simulink model "gm_sampleModel1839_sub_sub"  (R2023a)
settings: Solver=VariableStepAuto  StartTime=0.0  StopTime=10.0  RelTol=1e-3
libraries: hdlsllib x3, simulink x1
settings Model: Creator=user1  LastModifiedBy=user1
settings OptimizationCC: BlockReduction=off  ConditionallyExecuteInputs=off
settings DebuggingCC: InheritedTsInSrcMsg=none

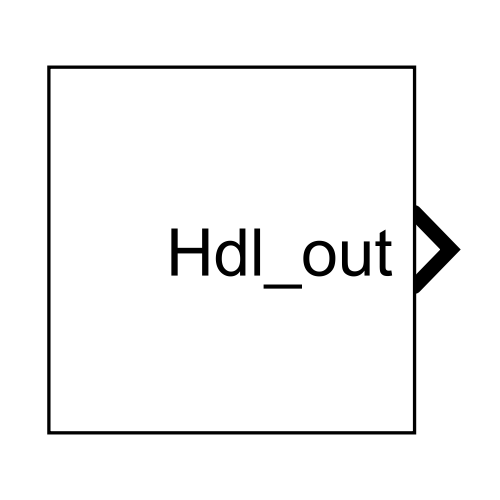
[thumbnail: Simulink's stored preview of the top-level diagram]
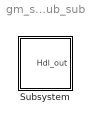
== system gm_sampleModel1839_sub_sub ==
  Subsystem : Subsystem

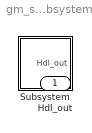
== system gm_sampleModel1839_sub_sub/Subsystem ==
  Subsystem : Subsystem
  Hdl_out : Outport  OutDataTypeStr=uint8

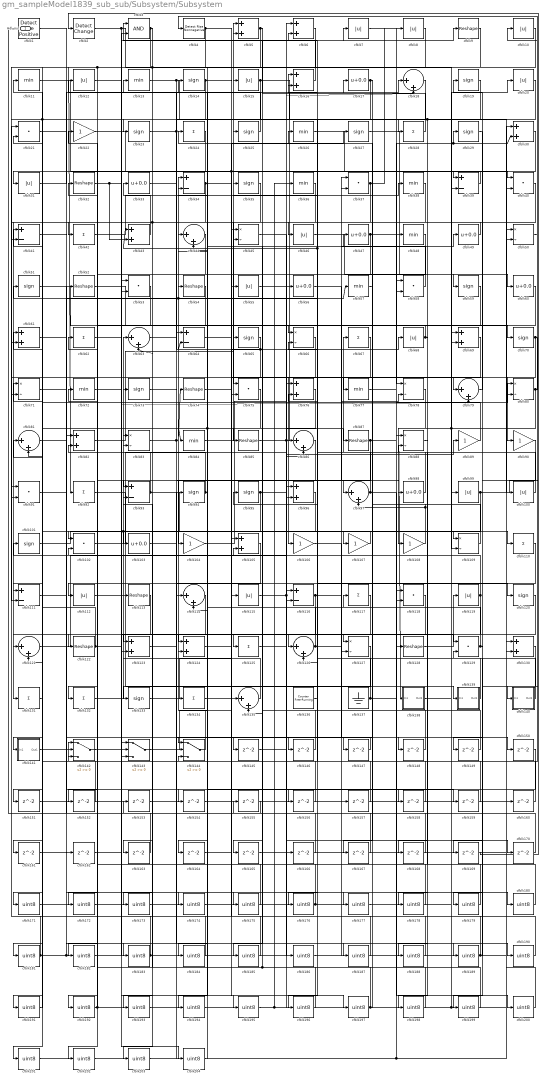
== system gm_sampleModel1839_sub_sub/Subsystem/Subsystem ==
  cfblk1 : hdlsllib/Logic and Bit Operations/Detect Rise Positive  vinit=0  OutDataTypeStr=uint8
  cfblk{7..8,10,12,15,20,31,46,55,68,99..100,112,115,119} (15 alike) : Abs  OutDataTypeStr=uint8  SaturateOnIntegerOverflow=off
  cfblk{14,19,23,25,27,29,35,51,59,65,70,73,94..95,101,120,133} (17 alike) : Signum
  cfblk{21,37,40,53,58,75,91,102,118,129} (10 alike) : DotProduct  OutDataTypeStr=uint8
  cfblk{17,33,47,49,56,60,98,103} (8 alike) : Bias  Bias=0.0  SaturateOnIntegerOverflow=off
  cfblk{22,89..90,104,106..108} (7 alike) : Gain  OutDataTypeStr=uint8
  cfblk{5..6,16,30,43,61,69,76,82,96,105,123..124,130} (14 alike) : Sum  OutDataTypeStr=uint8
  cfblk{45,50,66,71,78,80,83,88,109,127} (10 alike) : Product  Inputs=*/  OutDataTypeStr=uint8  RndMeth=Zero  SaturateOnIntegerOverflow=on
  cfblk{11,13,26,36,38,48,57,72,77,84} (10 alike) : MinMax  OutDataTypeStr=uint8
  cfblk{24,28,42,62,67,92,110,117,125,131..132,134} (12 alike) : Sum  Inputs=+  OutDataTypeStr=uint8
  cfblk{34,39,41,64,93,111,116} (7 alike) : Sum  Inputs=+-  OutDataTypeStr=uint8
  cfblk{9,32,52,54,74,85,87,113,122,128} (10 alike) : Reshape
  cfblk{18,44,63,79,81,86,97,114,121,126,135} (11 alike) : Sum  Inputs=|++  OutDataTypeStr=uint8
  cfblk136 : hdlsllib/Sources/Counter Free-Running  NumBits=16  tsamp=-1
  cfblk137 : Ground
  cfblk138 : Subsystem
      settings: LibrarySourceBlock=|
      | hdlsllib/Ports &
      | Subsystems/Subsystem
  cfblk139 : Subsystem
      settings: LibrarySourceBlock=|
      | hdlsllib/Ports &
      | Subsystems/Subsystem
  cfblk140 : Subsystem
      settings: LibrarySourceBlock=|
      | hdlsllib/Ports &
      | Subsystems/Subsystem
  cfblk141 : Subsystem
      settings: LibrarySourceBlock=|
      | hdlsllib/Ports &
      | Subsystems/Subsystem
  cfblk142 : Switch  OutDataTypeStr=uint8  SaturateOnIntegerOverflow=off  InputSameDT=off
  cfblk143 : Switch  OutDataTypeStr=uint8  SaturateOnIntegerOverflow=off  InputSameDT=off
  cfblk144 : Switch  OutDataTypeStr=uint8  SaturateOnIntegerOverflow=off  InputSameDT=off
  cfblk{145..170} (26 alike) : Delay  SampleTime=1
  cfblk{171..204} (34 alike) : DataTypeConversion  OutDataTypeStr=uint8  SaturateOnIntegerOverflow=off  RndMeth=Floor
  cfblk2 : simulink/Logic and Bit Operations/Detect Change  vinit=0  OutDataTypeStr=uint8
      settings: LibrarySourceBlock=|
      | hdlsllib/Logic and Bit
      | Operations/Detect
      | Change
  cfblk3 : Logic  AllPortsSameDT=off  OutDataTypeStr=boolean
  cfblk4 : hdlsllib/Logic and Bit Operations/Detect Rise Nonnegative  vinit=0  OutDataTypeStr=uint8
  Hdl_out : Outport  OutDataTypeStr=uint8
  wires:
  cfblk130/1 -> cfblk199/1
  cfblk128/1 -> cfblk119/1
  cfblk35/1 -> cfblk131/1
  cfblk70/1 -> cfblk140/1(In1), cfblk90/1
  cfblk126/1 -> cfblk78/2, cfblk101/1
  cfblk52/1 -> cfblk70/1
  cfblk21/1 -> cfblk183/1
  cfblk85/1 -> cfblk87/1, cfblk17/1
  cfblk68/1 -> cfblk168/1, cfblk66/1
  cfblk84/1 -> cfblk5/1
  cfblk40/1 -> cfblk75/1
  cfblk37/1 -> cfblk133/1, cfblk8/1
  cfblk22/1 -> cfblk39/1
  cfblk108/1 -> cfblk97/2, cfblk24/1
  cfblk115/1 -> cfblk170/1, cfblk18/2
  cfblk49/1 -> cfblk46/1
  cfblk50/1 -> cfblk4/1
  cfblk104/1 -> cfblk56/1
  cfblk95/1 -> cfblk89/1, cfblk103/1, cfblk111/1
  cfblk98/1 -> cfblk67/1
  cfblk144/1 -> cfblk34/1
  cfblk83/1 -> cfblk159/1, cfblk74/1
  cfblk4/1 -> cfblk180/1, cfblk173/1, cfblk42/1, cfblk92/1
  cfblk140/1(Out1) -> cfblk35/1
  cfblk16/1 -> cfblk3/1
  cfblk5/1 -> cfblk165/1, cfblk164/1
  cfblk132/1 -> cfblk63/1
  cfblk19/1 -> cfblk194/1, cfblk84/1
  cfblk87/1 -> cfblk104/1, cfblk30/2, cfblk29/1
  cfblk27/1 -> cfblk59/1
  cfblk72/1 -> cfblk195/1
  cfblk97/1 -> cfblk200/1, cfblk16/1
  cfblk92/1 -> cfblk139/1(In1)
  cfblk101/1 -> cfblk107/1
  cfblk66/1 -> cfblk85/1
  cfblk76/1 -> cfblk121/1
  cfblk73/1 -> cfblk120/1
  cfblk17/1 -> cfblk147/1, cfblk146/1
  cfblk42/1 -> cfblk38/1
  cfblk82/1 -> cfblk65/1
  cfblk135/1 -> cfblk73/1
  cfblk18/1 -> cfblk124/1
  cfblk133/1 -> cfblk55/1
  cfblk48/1 -> cfblk125/1
  cfblk109/1 -> cfblk25/1
  cfblk93/1 -> cfblk83/2, cfblk110/1
  cfblk69/1 -> cfblk111/2
  cfblk138/1(Out1) -> cfblk20/1
  cfblk65/1 -> cfblk91/2, cfblk64/2
  cfblk39/1 -> cfblk31/1
  cfblk116/1 -> cfblk143/3, cfblk49/1
  cfblk122/1 -> cfblk129/1, cfblk41/1
  cfblk36/1 -> cfblk41/2
  cfblk14/1 -> cfblk77/1, cfblk23/1
  cfblk47/1 -> cfblk152/1, cfblk80/2
  cfblk67/1 -> cfblk106/1
  cfblk43/1 -> cfblk33/1
  cfblk143/1 -> cfblk68/1
  cfblk64/1 -> cfblk126/1
  cfblk46/1 -> cfblk60/1
  cfblk59/1 -> cfblk123/1
  cfblk137/1 -> cfblk80/1, cfblk95/1
  cfblk6/1 -> cfblk144/1
  cfblk79/1 -> cfblk19/1
  cfblk119/1 -> cfblk161/1, cfblk83/1
  cfblk102/1 -> cfblk6/1
  cfblk94/1 -> cfblk44/2, cfblk32/1
  cfblk131/1 -> cfblk71/1
  cfblk99/1 -> cfblk191/1, cfblk142/1
  cfblk26/1 -> cfblk58/1
  cfblk51/1 -> cfblk116/1
  cfblk141/1(Out1) -> cfblk54/1, cfblk57/1
  cfblk80/1 -> cfblk10/1, cfblk109/2, cfblk138/1(In1)
  cfblk1/1 -> cfblk82/1
  cfblk25/1 -> cfblk13/1
  cfblk13/1 -> cfblk127/2, cfblk100/1
  cfblk3/1 -> cfblk203/1, cfblk61/2
  cfblk114/1 -> cfblk202/1
  cfblk81/1 -> cfblk189/1
  cfblk23/1 -> cfblk28/1, cfblk109/1
  cfblk139/1(Out1) -> cfblk51/1
  cfblk107/1 -> cfblk102/1
  cfblk32/1 -> cfblk43/2, cfblk127/1
  cfblk136/1 -> cfblk26/1
  cfblk38/1 -> cfblk132/1
  cfblk78/1 -> cfblk108/1
  cfblk96/1 -> cfblk135/2
  cfblk15/1 -> cfblk53/2, cfblk99/1
  cfblk11/1 -> cfblk78/1, cfblk115/1
  cfblk129/1 -> cfblk179/1, cfblk12/1
  cfblk121/1 -> cfblk96/2
  cfblk74/1 -> cfblk27/1
  cfblk134/1 -> cfblk197/1
  cfblk113/1 -> cfblk181/1
  cfblk7/1 -> cfblk40/1
  cfblk10/1 -> cfblk201/1, cfblk63/2
  cfblk86/1 -> cfblk192/1
  cfblk56/1 -> cfblk98/1
  cfblk55/1 -> cfblk7/1
  cfblk2/1 -> cfblk79/2, cfblk69/2
  cfblk117/1 -> cfblk176/1
  cfblk124/1 -> cfblk75/2
  cfblk33/1 -> cfblk97/1
  cfblk100/1 -> cfblk16/2, cfblk43/1
  cfblk31/1 -> cfblk15/1
  cfblk34/1 -> cfblk79/1, cfblk193/1, cfblk143/2
  cfblk63/1 -> cfblk18/1
  cfblk44/1 -> cfblk93/1
  cfblk20/1 -> cfblk188/1, cfblk141/1(In1), cfblk71/2
  cfblk8/1 -> cfblk122/1
  cfblk77/1 -> cfblk48/1
  cfblk58/1 -> cfblk14/1
  cfblk24/1 -> cfblk112/1
  cfblk89/1 -> cfblk61/1
  cfblk54/1 -> cfblk123/2
  cfblk28/1 -> cfblk5/2
  cfblk142/1 -> cfblk9/1
  cfblk111/1 -> cfblk52/1
  cfblk60/1 -> cfblk145/1
  cfblk145/1 -> cfblk116/2
  cfblk146/1 -> cfblk64/1
  cfblk147/1 -> cfblk144/2
  cfblk106/1 -> cfblk148/1
  cfblk148/1 -> cfblk66/2
  cfblk29/1 -> cfblk149/1
  cfblk149/1 -> cfblk102/2
  cfblk41/1 -> cfblk150/1
  cfblk75/1 -> cfblk151/1
  cfblk151/1 -> cfblk96/1
  cfblk152/1 -> cfblk121/2
  cfblk153/1 -> cfblk37/1
  cfblk12/1 -> cfblk154/1
  cfblk154/1 -> cfblk50/2
  cfblk155/1 -> cfblk1/1
  cfblk110/1 -> cfblk156/1
  cfblk156/1 -> cfblk34/2
  cfblk157/1 -> cfblk76/2
  cfblk91/1 -> cfblk158/1
  cfblk158/1 -> cfblk105/2
  cfblk159/1 -> cfblk126/2
  cfblk160/1 -> cfblk6/2
  cfblk161/1 -> cfblk3/2
  cfblk61/1 -> cfblk162/1
  cfblk162/1 -> cfblk143/1
  cfblk127/1 -> cfblk163/1
  cfblk163/1 -> cfblk142/3
  cfblk164/1 -> cfblk135/1
  cfblk165/1 -> cfblk30/1
  cfblk125/1 -> cfblk166/1
  cfblk166/1 -> cfblk82/2
  cfblk57/1 -> cfblk167/1
  cfblk167/1 -> cfblk142/2
  cfblk168/1 -> cfblk144/3
  cfblk90/1 -> cfblk169/1
  cfblk169/1 -> cfblk2/1
  cfblk170/1 -> cfblk11/1
  cfblk118/1 -> cfblk171/1
  cfblk171/1 -> cfblk94/1
  cfblk53/1 -> cfblk172/1
  cfblk172/1 -> cfblk118/1
  cfblk173/1 -> cfblk118/2
  cfblk62/1 -> cfblk174/1
  cfblk174/1 -> cfblk69/1
  cfblk103/1 -> cfblk175/1
  cfblk175/1 -> cfblk62/1
  cfblk176/1 -> cfblk58/2, cfblk44/1
  cfblk71/1 -> cfblk177/1
  cfblk177/1 -> cfblk117/1
  cfblk88/1 -> cfblk178/1
  cfblk178/1 -> cfblk153/1
  cfblk179/1 -> cfblk88/1
  cfblk180/1 -> cfblk88/2
  cfblk181/1 -> cfblk91/1, cfblk187/1, cfblk157/1
  cfblk105/1 -> cfblk182/1
  cfblk182/1 -> cfblk113/1
  cfblk183/1 -> cfblk50/1, cfblk53/1
  cfblk150/1 -> cfblk184/1
  cfblk184/1 -> cfblk21/1
  cfblk9/1 -> cfblk185/1
  cfblk185/1 -> cfblk21/2
  cfblk45/1 -> cfblk186/1
  cfblk186/1 -> cfblk37/2
  cfblk187/1 -> cfblk45/1
  cfblk188/1 -> cfblk45/2
  cfblk189/1 -> cfblk105/1, cfblk129/2
  cfblk123/1 -> cfblk190/1
  cfblk190/1 -> cfblk81/1
  cfblk191/1 -> cfblk81/2
  cfblk192/1 -> cfblk22/1, cfblk39/2, cfblk40/2
  cfblk193/1 -> cfblk86/1
  cfblk194/1 -> cfblk86/2
  cfblk195/1 -> cfblk36/1, cfblk76/1
  cfblk30/1 -> cfblk196/1
  cfblk196/1 -> cfblk72/1
  cfblk197/1 -> cfblk124/2, cfblk47/1
  cfblk120/1 -> cfblk198/1
  cfblk198/1 -> cfblk134/1
  cfblk199/1 -> cfblk93/2, cfblk155/1
  cfblk200/1 -> cfblk130/1
  cfblk201/1 -> cfblk130/2
  cfblk202/1 -> cfblk128/1, cfblk160/1
  cfblk203/1 -> cfblk114/1
  cfblk112/1 -> cfblk204/1
  cfblk204/1 -> cfblk114/2

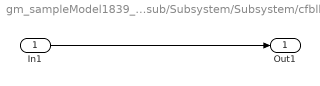
== system gm_sampleModel1839_sub_sub/Subsystem/Subsystem/cfblk138 ==
  In1 : Inport
  Out1 : Outport
  wires:
  In1/1 -> Out1/1

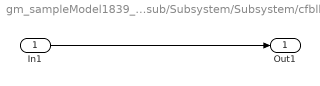
== system gm_sampleModel1839_sub_sub/Subsystem/Subsystem/cfblk139 ==
  In1 : Inport
  Out1 : Outport
  wires:
  In1/1 -> Out1/1

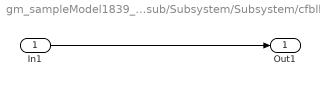
== system gm_sampleModel1839_sub_sub/Subsystem/Subsystem/cfblk140 ==
  In1 : Inport
  Out1 : Outport
  wires:
  In1/1 -> Out1/1

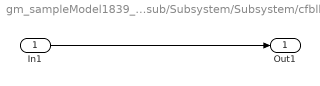
== system gm_sampleModel1839_sub_sub/Subsystem/Subsystem/cfblk141 ==
  In1 : Inport
  Out1 : Outport
  wires:
  In1/1 -> Out1/1
